simulink model "understandingof_sumof_sinewaves"  (R2024b)
settings: Solver=VariableStepAuto  StartTime=0.0  StopTime=10.0  MaxStep=0.01  RelTol=1e-3
settings Model: Creator=admin  LastModifiedBy=admin

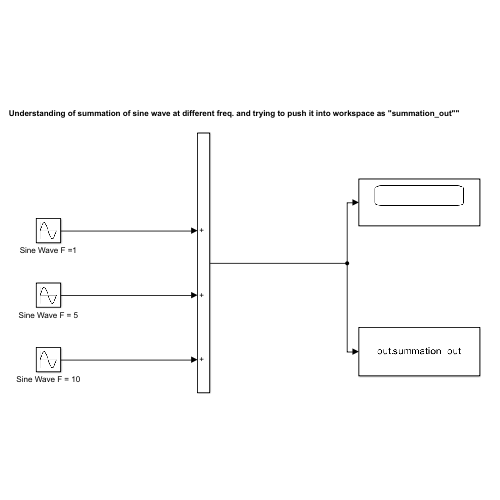
[thumbnail: Simulink's stored preview of the top-level diagram]
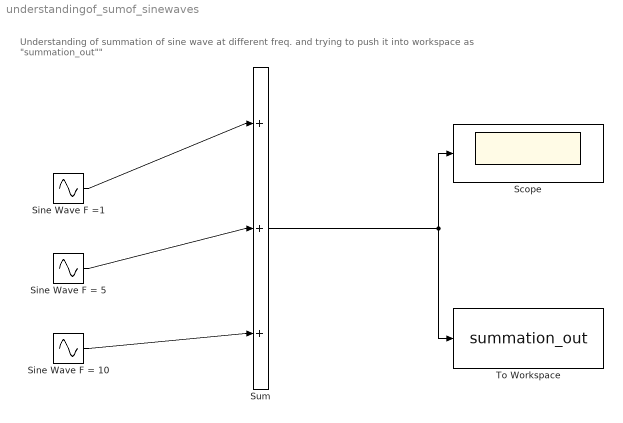
== system understandingof_sumof_sinewaves ==
  note: Understanding of summation of sine wave at different freq. and trying to push it into workspace as "summation_out""
  Scope : Scope
  Sine Wave F = 10 : Sin  Frequency=10  SampleTime=0
  Sine Wave F = 5 : Sin  Frequency=5  SampleTime=0
  Sine Wave F =1 : Sin  SampleTime=0
  Sum : Sum  Inputs=|+++
  To Workspace : ToWorkspace  VariableName=summation_out  SaveFormat=Timeseries  SampleTime=-1
  wires:
  Sum/1 -> To Workspace/1, Scope/1
  Sine Wave F =1/1 -> Sum/1
  Sine Wave F = 5/1 -> Sum/2
  Sine Wave F = 10/1 -> Sum/3
